simulink model "ss1"  (R2013a)
settings: Solver=ode3  StartTime=0.0  StopTime=10  FixedStep=T  RelTol=1e-3
values from neighbouring files (symbols this model uses):
  A = [0 1; 0 0]    [ss1_init.m]    (also in ss512_init.m = [0 0 1 0; ss51_init.m = [0 0 1 0)
  B = [0; 1]    [ss1_init.m]    (also in ss512_init.m = [0; 0; 0; 1]; ss51_init.m = [0; 0; 0; 1])
  C = eye(2)    [ss1_init.m]    (also in ss512_init.m = eye(n); ss51_init.m = eye(n))
  D = [0; 0]    [ss1_init.m]    (also in ss512_init.m = zeros([n 1]); ss51_init.m = zeros([n 1]))
  H = [1 0]    [ex8_init.m]    (also in ss512_init.m = [1 0 0 0])
  K = acker(Phi, Gam, p)    [ex8_init.m]    (also in myacker.m = en*(W\alpha); ss1_init.m = myacker(Phi, Gamma, z))
  Phi = [1 T; 0 1]    [ex8_init.m]
  T = 0.1    [ex8_init.m]    (also in ss1_init.m; ss512_init.m = 0.4; ss51_init.m = 0.4)
  x1 = [1; 0]    [ex8_init.m]    (also in ss1_init.m = [1; 1]; ss512_init.m = [1; 0; 0; 0]; ss51_init.m = [1; 0; 0; 0])
undefined symbols (not defined in the file or in its folder): G, Gamma
settings Model: Creator=jmahler  LastModifiedBy=jmahler

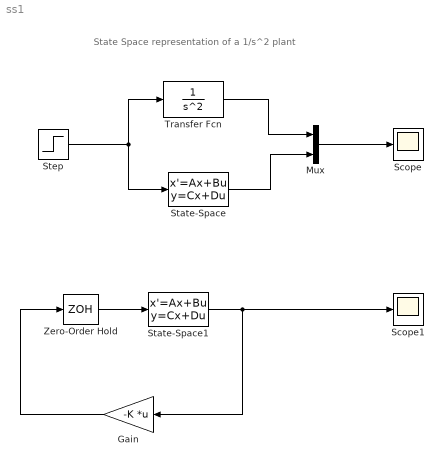
== system ss1 ==
  note: State Space representation of a 1/s^2 plant
  Gain : Gain  Gain=-K  Multiplication=Matrix(K*u)
  Mux : Mux  Inputs=2
  Scope : Scope
  Scope1 : Scope
  State-Space : StateSpace  A=A  B=B  C=C  D=D  X0=x1
  State-Space1 : StateSpace  A=Phi  B=Gamma  C=H  D=G  X0=x1
  Step : Step  SampleTime=0
  Transfer Fcn : TransferFcn  Denominator=[1 0 0]
  Zero-Order Hold : ZeroOrderHold  SampleTime=T
  wires:
  Step/1 -> State-Space/1, Transfer Fcn/1
  Transfer Fcn/1 -> Mux/1
  State-Space/1 -> Mux/2
  Mux/1 -> Scope/1
  Gain/1 -> Zero-Order Hold/1
  Zero-Order Hold/1 -> State-Space1/1
  State-Space1/1 -> Gain/1, Scope1/1
